simulink model "untitled"  (Simulink 7.3)
settings: Solver=ode45  StartTime=0.0  StopTime=10.0  RelTol=1e-3
values from neighbouring files (symbols this model uses):
  m = 10    [CASEfinder.m]    (also in Example_2ODE_system.m = 9; Example_check_mLyapunov.m; Example_check_mriccati.m)
  R = 100    [Sensitivity_Practice.m]
  w = w_rand_3    [CASEfinder.m]    (also in Example_check_mLyapunov.m; Example_check_mriccati.m; Example_in_Kang_paper.m = 1*rand(length([0:Ts:t_final]),size(Bn,2))'; Road_noise.m = zeros(4,length([0 :Ts: finite_time_of_DOC])))
undefined symbols (not defined in the file or in its folder): DiscIntNeverNeededParam, g, h, Izz, l, lf, lr, ms, mus
settings Model: Creator=SH  LastModifiedBy=SH

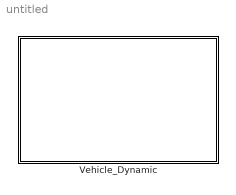
== system untitled ==
  Vehicle_Dynamic : Subsystem
      mask Display: image(imread('V1.jpg'))

== system untitled/Vehicle_Dynamic ==
  Global_position : Subsystem
  Lateral_Dynamic : Subsystem
  Longitudinal_Dynamic : Subsystem
  SlipRatio&SlipAngle : Subsystem
  TireForce : Subsystem
  VerticalForce : Subsystem
  Yaw_Dynamic : Subsystem

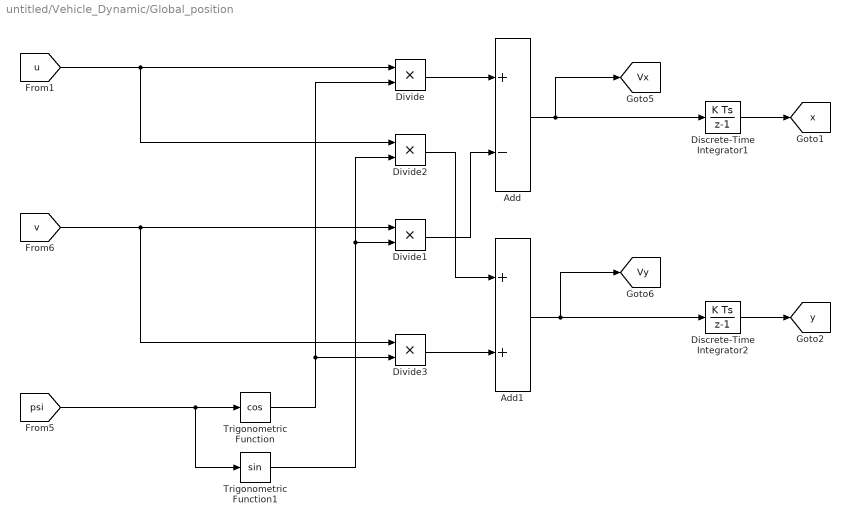
== system untitled/Vehicle_Dynamic/Global_position ==
  Add : Sum  Inputs=+-  OutDataType=fixdt(1, 16)  OutScaling=2^-10
  Add1 : Sum  OutDataType=fixdt(1, 16)  OutScaling=2^-10
  Discrete-Time Integrator1 : DiscreteIntegrator  SampleTime=-1  OutDataType=fixdt(1, 16)  OutScaling=2^0  ICPrevOutput=DiscIntNeverNeededParam  ICPrevScaledInput=DiscIntNeverNeededParam
  Discrete-Time Integrator2 : DiscreteIntegrator  SampleTime=-1  OutDataType=fixdt(1, 16)  OutScaling=2^0  ICPrevOutput=DiscIntNeverNeededParam  ICPrevScaledInput=DiscIntNeverNeededParam
  Divide{,1..3} (4 alike) : Product  Inputs=**  OutDataType=fixdt(1, 16)  OutScaling=2^-10
  Trigonometric Function : Trigonometry  Operator=cos
  Trigonometric Function1 : Trigonometry
  tag scope: Vx=global, Vy=global, x=global, y=global
  wires:
  Add1/1 -> [Vy], Discrete-Time Integrator2/1
  Divide3/1 -> Add1/2
  Divide2/1 -> Add1/1
  Divide1/1 -> Add/2
  Divide/1 -> Add/1
  [v] -> Divide3/1, Divide1/1
  [u] -> Divide2/1, Divide/1
  Discrete-Time Integrator2/1 -> [y]
  Trigonometric Function/1 -> Divide/2, Divide3/2
  Trigonometric Function1/1 -> Divide1/2, Divide2/2
  [psi] -> Trigonometric Function/1, Trigonometric Function1/1
  Discrete-Time Integrator1/1 -> [x]
  Add/1 -> [Vx], Discrete-Time Integrator1/1

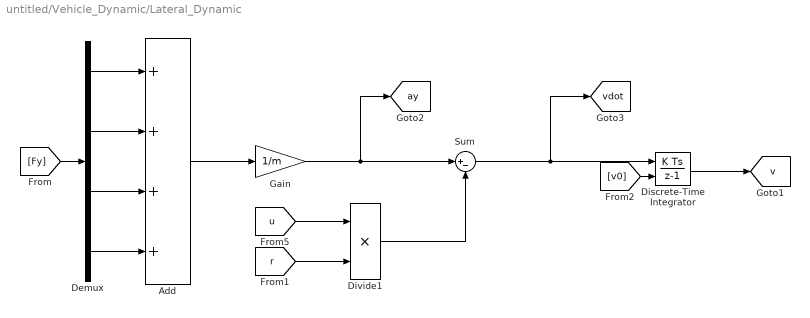
== system untitled/Vehicle_Dynamic/Lateral_Dynamic ==
  Add : Sum  Inputs=++++  OutDataType=fixdt(1, 16)  OutScaling=2^-10
  Demux : Demux
  Discrete-Time Integrator : DiscreteIntegrator  InitialConditionSource=external  SampleTime=-1  OutDataType=fixdt(1, 16)  OutScaling=2^0  ICPrevOutput=DiscIntNeverNeededParam  ICPrevScaledInput=DiscIntNeverNeededParam
  Divide1 : Product  Inputs=**  OutDataType=fixdt(1, 16)  OutScaling=2^-10
  Gain : Gain  Gain=1/m  ParameterDataType=fixdt(1, 16)  ParameterScaling=2^0  OutDataType=fixdt(1, 16)  OutScaling=2^0
  Sum : Sum  Inputs=|+-  OutDataType=fixdt(1, 16)  OutScaling=2^0
  tag scope: ay=global, v=global, vdot=global
  wires:
  Discrete-Time Integrator/1 -> [v]
  [u] -> Divide1/1
  Sum/1 -> Discrete-Time Integrator/1, [vdot]
  Add/1 -> Gain/1
  Gain/1 -> [ay], Sum/1
  [r] -> Divide1/2
  Demux/4 -> Add/4
  Demux/3 -> Add/3
  Demux/2 -> Add/2
  Demux/1 -> Add/1
  [Fy] -> Demux/1
  [v0] -> Discrete-Time Integrator/2
  Divide1/1 -> Sum/2

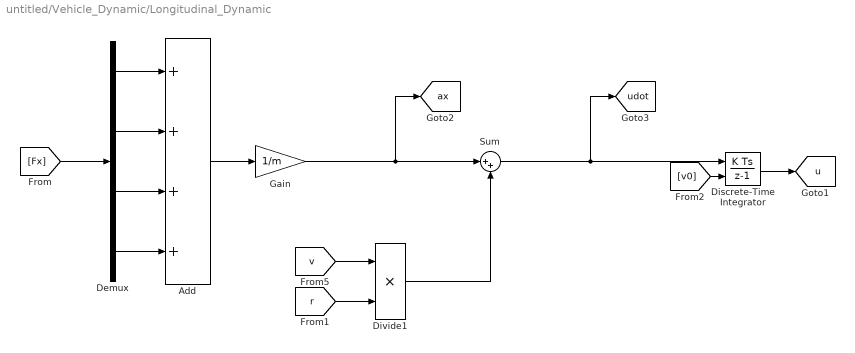
== system untitled/Vehicle_Dynamic/Longitudinal_Dynamic ==
  Add : Sum  Inputs=++++  OutDataType=fixdt(1, 16)  OutScaling=2^-10
  Demux : Demux
  Discrete-Time Integrator : DiscreteIntegrator  InitialConditionSource=external  SampleTime=-1  OutDataType=fixdt(1, 16)  OutScaling=2^0  ICPrevOutput=DiscIntNeverNeededParam  ICPrevScaledInput=DiscIntNeverNeededParam
  Divide1 : Product  Inputs=**  OutDataType=fixdt(1, 16)  OutScaling=2^-10
  Gain : Gain  Gain=1/m  ParameterDataType=fixdt(1, 16)  ParameterScaling=2^0  OutDataType=fixdt(1, 16)  OutScaling=2^0
  Sum : Sum  Inputs=|++  OutDataType=fixdt(1, 16)  OutScaling=2^0
  tag scope: ax=global, u=global, udot=global
  wires:
  Discrete-Time Integrator/1 -> [u]
  Sum/1 -> Discrete-Time Integrator/1, [udot]
  [v] -> Divide1/1
  Add/1 -> Gain/1
  Gain/1 -> [ax], Sum/1
  Demux/4 -> Add/4
  Demux/3 -> Add/3
  Demux/2 -> Add/2
  Demux/1 -> Add/1
  [Fx] -> Demux/1
  [r] -> Divide1/2
  [v0] -> Discrete-Time Integrator/2
  Divide1/1 -> Sum/2

== system untitled/Vehicle_Dynamic/SlipRatio&SlipAngle ==
  Slip_angle : Subsystem
  Slip_ratio : Subsystem
  Tire_Longitudinal_Velocity : Subsystem
  Velocity_at_each_wheel : Subsystem

== system untitled/Vehicle_Dynamic/TireForce ==
  FL : Subsystem
  FR : Subsystem
  RL : Subsystem
  RR : Subsystem

== system untitled/Vehicle_Dynamic/VerticalForce ==
  VerticalForce_FL : Subsystem
  VerticalForce_FR : Subsystem
  VerticalForce_RL : Subsystem
  VerticalForce_RR : Subsystem

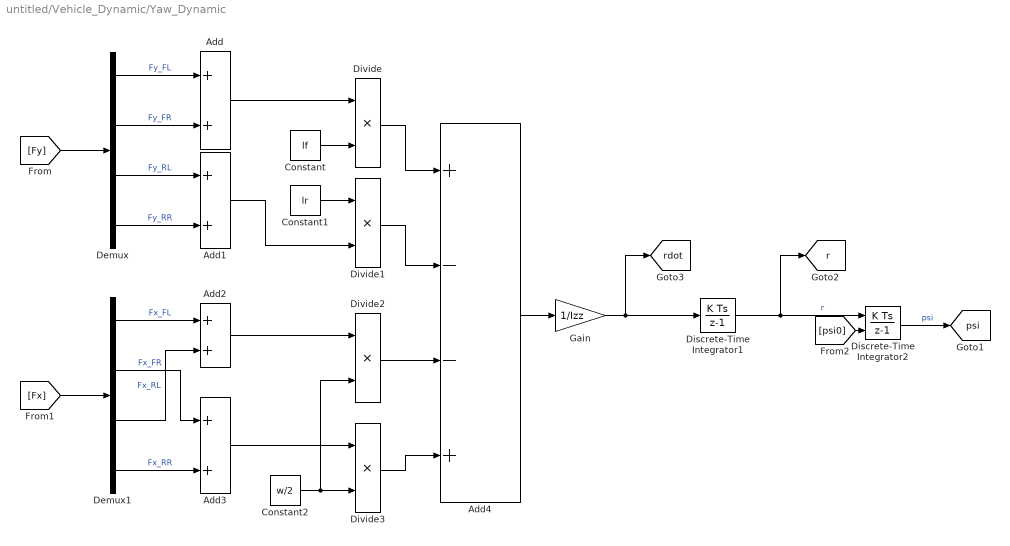
== system untitled/Vehicle_Dynamic/Yaw_Dynamic ==
  Add{,1..3} (4 alike) : Sum  OutDataType=fixdt(1, 16)  OutScaling=2^-10
  Add4 : Sum  Inputs=+--+  OutDataType=fixdt(1, 16)  OutScaling=2^-10
  Constant : Constant  Value=lf  OutDataType=fixdt(1, 16)  OutScaling=2^0
  Constant1 : Constant  Value=lr  OutDataType=fixdt(1, 16)  OutScaling=2^0
  Constant2 : Constant  Value=w/2  OutDataType=fixdt(1, 16)  OutScaling=2^0
  Demux : Demux
  Demux1 : Demux
  Discrete-Time Integrator1 : DiscreteIntegrator  SampleTime=-1  OutDataType=fixdt(1, 16)  OutScaling=2^0  ICPrevOutput=DiscIntNeverNeededParam  ICPrevScaledInput=DiscIntNeverNeededParam
  Discrete-Time Integrator2 : DiscreteIntegrator  InitialConditionSource=external  SampleTime=-1  OutDataType=fixdt(1, 16)  OutScaling=2^0  ICPrevOutput=DiscIntNeverNeededParam  ICPrevScaledInput=DiscIntNeverNeededParam
  Divide{,1..3} (4 alike) : Product  Inputs=**  OutDataType=fixdt(1, 16)  OutScaling=2^-10
  Gain : Gain  Gain=1/Izz  ParameterDataType=fixdt(1, 16)  ParameterScaling=2^0  OutDataType=fixdt(1, 16)  OutScaling=2^0
  tag scope: psi=global, r=global, rdot=global
  wires:
  Add/1 -> Divide/1
  Gain/1 -> Discrete-Time Integrator1/1, [rdot]
  Discrete-Time Integrator1/1 -> Discrete-Time Integrator2/1, [r]  "r"
  Discrete-Time Integrator2/1 -> [psi]  "psi"
  Divide/1 -> Add4/1
  Constant/1 -> Divide/2
  Divide2/1 -> Add4/3
  Divide1/1 -> Add4/2
  Add4/1 -> Gain/1
  Demux/2 -> Add/2  "Fy_FR"
  Demux/1 -> Add/1  "Fy_FL"
  [Fy] -> Demux/1
  [Fx] -> Demux1/1
  [psi0] -> Discrete-Time Integrator2/2
  Demux/3 -> Add1/1  "Fy_RL"
  Demux/4 -> Add1/2  "Fy_RR"
  Constant1/1 -> Divide1/1
  Add1/1 -> Divide1/2
  Divide3/1 -> Add4/4
  Demux1/1 -> Add2/1  "Fx_FL"
  Demux1/4 -> Add3/2  "Fx_RR"
  Add2/1 -> Divide2/1
  Demux1/3 -> Add2/2  "Fx_RL"
  Demux1/2 -> Add3/1  "Fx_FR"
  Add3/1 -> Divide3/1
  Constant2/1 -> Divide3/2, Divide2/2

== system untitled/Vehicle_Dynamic/SlipRatio&SlipAngle/Slip_angle ==
  SlipAngle_FL : Subsystem
  SlipAngle_FR : Subsystem
  SlipAngle_RL : Subsystem
  SlipAngle_RR : Subsystem

== system untitled/Vehicle_Dynamic/SlipRatio&SlipAngle/Slip_ratio ==
  Slipratio_FL : Subsystem
  Slipratio_FR : Subsystem
  Slipratio_RL : Subsystem
  Slipratio_RR : Subsystem

== system untitled/Vehicle_Dynamic/SlipRatio&SlipAngle/Tire_Longitudinal_Velocity ==
  uu_FL : Subsystem
  uu_FR : Subsystem
  uu_RL : Subsystem
  uu_RR : Subsystem

== system untitled/Vehicle_Dynamic/SlipRatio&SlipAngle/Velocity_at_each_wheel ==
  uv_FL : Subsystem
  uv_FR : Subsystem
  uv_RL : Subsystem
  uv_RR : Subsystem

== system untitled/Vehicle_Dynamic/TireForce/FL ==
  SideForce : Subsystem
  TractionForce : Subsystem

== system untitled/Vehicle_Dynamic/TireForce/FR ==
  SideForce : Subsystem
  TractionForce : Subsystem

== system untitled/Vehicle_Dynamic/TireForce/RL ==
  SideForce : Subsystem
  TractionForce : Subsystem

== system untitled/Vehicle_Dynamic/TireForce/RR ==
  SideForce : Subsystem
  TractionForce : Subsystem

== system untitled/Vehicle_Dynamic/VerticalForce/VerticalForce_FL ==
  C.G.Effect : Subsystem
  PitchEffect : Subsystem
  Sum : Sum  Inputs=++-  OutDataType=fixdt(1, 16)  OutScaling=2^0
  TireWeight : Subsystem
  tag scope: Fz_FL=global
  wires:
  Sum/1 -> [Fz_FL]
  TireWeight/1(Out1) -> Sum/1
  C.G.Effect/1(Out1) -> Sum/2
  PitchEffect/1(Out1) -> Sum/3

== system untitled/Vehicle_Dynamic/VerticalForce/VerticalForce_FR ==
  C.G.Effect : Subsystem
  PitchEffect : Subsystem
  Sum : Sum  Inputs=++-  OutDataType=fixdt(1, 16)  OutScaling=2^0
  TireWeight : Subsystem
  tag scope: Fz_FR=global
  wires:
  Sum/1 -> [Fz_FR]
  TireWeight/1(Out1) -> Sum/1
  C.G.Effect/1(Out1) -> Sum/2
  PitchEffect/1(Out1) -> Sum/3

== system untitled/Vehicle_Dynamic/VerticalForce/VerticalForce_RL ==
  C.G.Effect : Subsystem
  PitchEffect : Subsystem
  Sum : Sum  Inputs=+++  OutDataType=fixdt(1, 16)  OutScaling=2^0
  TireWeight : Subsystem
  tag scope: Fz_RL=global
  wires:
  PitchEffect/1(Out1) -> Sum/3
  C.G.Effect/1(Out1) -> Sum/2
  TireWeight/1(Out1) -> Sum/1
  Sum/1 -> [Fz_RL]

== system untitled/Vehicle_Dynamic/VerticalForce/VerticalForce_RR ==
  C.G.Effect : Subsystem
  PitchEffect : Subsystem
  Sum : Sum  Inputs=+++  OutDataType=fixdt(1, 16)  OutScaling=2^0
  TireWeight : Subsystem
  tag scope: Fz_RR=global
  wires:
  PitchEffect/1(Out1) -> Sum/3
  C.G.Effect/1(Out1) -> Sum/2
  TireWeight/1(Out1) -> Sum/1
  Sum/1 -> [Fz_RR]

== system untitled/Vehicle_Dynamic/SlipRatio&SlipAngle/Slip_angle/SlipAngle_FL ==
  Gain : Gain  Gain=pi/180  ParameterDataType=fixdt(1, 16)  ParameterScaling=2^0  OutDataType=fixdt(1, 16)  OutScaling=2^0
  Sum : Sum  Inputs=|+-  OutDataType=fixdt(1, 16)  OutScaling=2^0
  Trigonometric Function : Trigonometry  Operator=atan2
  tag scope: slipA_FL=global
  wires:
  [SA_FL] -> Gain/1
  [u_FL] -> Trigonometric Function/2
  [v_FL] -> Trigonometric Function/1
  Trigonometric Function/1 -> Sum/2
  Gain/1 -> Sum/1
  Sum/1 -> [slipA_FL]

== system untitled/Vehicle_Dynamic/SlipRatio&SlipAngle/Slip_angle/SlipAngle_FR ==
  Gain : Gain  Gain=pi/180  ParameterDataType=fixdt(1, 16)  ParameterScaling=2^0  OutDataType=fixdt(1, 16)  OutScaling=2^0
  Sum : Sum  Inputs=|+-  OutDataType=fixdt(1, 16)  OutScaling=2^0
  Trigonometric Function : Trigonometry  Operator=atan2
  tag scope: slipA_FR=global
  wires:
  Sum/1 -> [slipA_FR]
  Gain/1 -> Sum/1
  Trigonometric Function/1 -> Sum/2
  [v_FR] -> Trigonometric Function/1
  [u_FR] -> Trigonometric Function/2
  [SA_FR] -> Gain/1

== system untitled/Vehicle_Dynamic/SlipRatio&SlipAngle/Slip_angle/SlipAngle_RL ==
  Gain : Gain  Gain=pi/180  ParameterDataType=fixdt(1, 16)  ParameterScaling=2^0  OutDataType=fixdt(1, 16)  OutScaling=2^0
  Sum : Sum  Inputs=|+-  OutDataType=fixdt(1, 16)  OutScaling=2^0
  Trigonometric Function : Trigonometry  Operator=atan2
  tag scope: slipA_RL=global
  wires:
  [SA_RL] -> Gain/1
  [u_RL] -> Trigonometric Function/2
  [v_RL] -> Trigonometric Function/1
  Trigonometric Function/1 -> Sum/2
  Gain/1 -> Sum/1
  Sum/1 -> [slipA_RL]

== system untitled/Vehicle_Dynamic/SlipRatio&SlipAngle/Slip_angle/SlipAngle_RR ==
  Gain : Gain  Gain=pi/180  ParameterDataType=fixdt(1, 16)  ParameterScaling=2^0  OutDataType=fixdt(1, 16)  OutScaling=2^0
  Sum : Sum  Inputs=|+-  OutDataType=fixdt(1, 16)  OutScaling=2^0
  Trigonometric Function : Trigonometry  Operator=atan2
  tag scope: slipA_RR=global
  wires:
  Sum/1 -> [slipA_RR]
  Gain/1 -> Sum/1
  Trigonometric Function/1 -> Sum/2
  [v_RR] -> Trigonometric Function/1
  [u_RR] -> Trigonometric Function/2
  [SA_RR] -> Gain/1

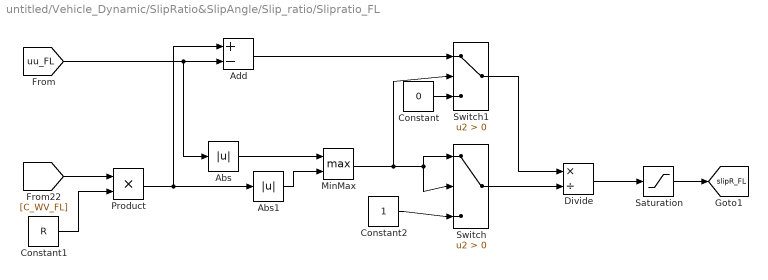
== system untitled/Vehicle_Dynamic/SlipRatio&SlipAngle/Slip_ratio/Slipratio_FL ==
  Abs : Abs  OutDataType=fixdt(1, 16)  OutScaling=2^0
  Abs1 : Abs  OutDataType=fixdt(1, 16)  OutScaling=2^0
  Add : Sum  Inputs=+-  OutDataType=fixdt(1, 16)  OutScaling=2^-10
  Constant : Constant  Value=0  OutDataType=fixdt(1, 16)  OutScaling=2^0
  Constant1 : Constant  Value=R  OutDataType=fixdt(1, 16)  OutScaling=2^0
  Constant2 : Constant  OutDataType=fixdt(1, 16)  OutScaling=2^0
  Divide : Product  Inputs=*/  OutDataType=fixdt(1, 16)  OutScaling=2^-10
  MinMax : MinMax  Function=max  Inputs=2  OutDataType=fixdt(1, 16)  OutScaling=2^0
  Product : Product  OutDataType=fixdt(1, 16)  OutScaling=2^0  RndMeth=Zero
  Saturation : Saturate  UpperLimit=1  LowerLimit=-1  OutDataType=fixdt(1, 16)  OutScaling=2^0
  Switch : Switch  Criteria=u2 > Threshold  OutDataType=fixdt(1, 16)  OutScaling=2^0
  Switch1 : Switch  Criteria=u2 > Threshold  OutDataType=fixdt(1, 16)  OutScaling=2^0
  tag scope: slipR_FL=global
  wires:
  [C_WV_FL] -> Product/1
  Constant1/1 -> Product/2
  Product/1 -> Add/1, Abs1/1
  [uu_FL] -> Add/2, Abs/1
  MinMax/1 -> Switch1/2, Switch/2, Switch/1
  Switch/1 -> Divide/2
  Abs/1 -> MinMax/1
  Abs1/1 -> MinMax/2
  Add/1 -> Switch1/1
  Switch1/1 -> Divide/1
  Constant/1 -> Switch1/3
  Constant2/1 -> Switch/3
  Divide/1 -> Saturation/1
  Saturation/1 -> [slipR_FL]

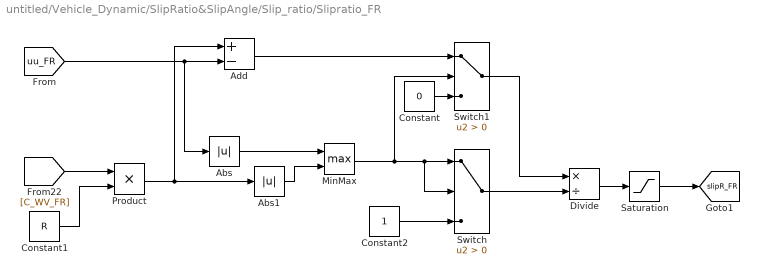
== system untitled/Vehicle_Dynamic/SlipRatio&SlipAngle/Slip_ratio/Slipratio_FR ==
  Abs : Abs  OutDataType=fixdt(1, 16)  OutScaling=2^0
  Abs1 : Abs  OutDataType=fixdt(1, 16)  OutScaling=2^0
  Add : Sum  Inputs=+-  OutDataType=fixdt(1, 16)  OutScaling=2^-10
  Constant : Constant  Value=0  OutDataType=fixdt(1, 16)  OutScaling=2^0
  Constant1 : Constant  Value=R  OutDataType=fixdt(1, 16)  OutScaling=2^0
  Constant2 : Constant  OutDataType=fixdt(1, 16)  OutScaling=2^0
  Divide : Product  Inputs=*/  OutDataType=fixdt(1, 16)  OutScaling=2^-10
  MinMax : MinMax  Function=max  Inputs=2  OutDataType=fixdt(1, 16)  OutScaling=2^0
  Product : Product  OutDataType=fixdt(1, 16)  OutScaling=2^0  RndMeth=Zero
  Saturation : Saturate  UpperLimit=1  LowerLimit=-1  OutDataType=fixdt(1, 16)  OutScaling=2^0
  Switch : Switch  Criteria=u2 > Threshold  OutDataType=fixdt(1, 16)  OutScaling=2^0
  Switch1 : Switch  Criteria=u2 > Threshold  OutDataType=fixdt(1, 16)  OutScaling=2^0
  tag scope: slipR_FR=global
  wires:
  Divide/1 -> Saturation/1
  Constant2/1 -> Switch/3
  Constant/1 -> Switch1/3
  Switch1/1 -> Divide/1
  Add/1 -> Switch1/1
  Abs1/1 -> MinMax/2
  Abs/1 -> MinMax/1
  Switch/1 -> Divide/2
  MinMax/1 -> Switch/1, Switch/2, Switch1/2
  [uu_FR] -> Abs/1, Add/2
  Product/1 -> Abs1/1, Add/1
  Constant1/1 -> Product/2
  [C_WV_FR] -> Product/1
  Saturation/1 -> [slipR_FR]

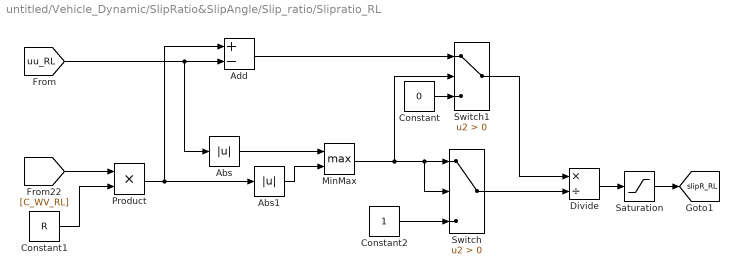
== system untitled/Vehicle_Dynamic/SlipRatio&SlipAngle/Slip_ratio/Slipratio_RL ==
  Abs : Abs  OutDataType=fixdt(1, 16)  OutScaling=2^0
  Abs1 : Abs  OutDataType=fixdt(1, 16)  OutScaling=2^0
  Add : Sum  Inputs=+-  OutDataType=fixdt(1, 16)  OutScaling=2^-10
  Constant : Constant  Value=0  OutDataType=fixdt(1, 16)  OutScaling=2^0
  Constant1 : Constant  Value=R  OutDataType=fixdt(1, 16)  OutScaling=2^0
  Constant2 : Constant  OutDataType=fixdt(1, 16)  OutScaling=2^0
  Divide : Product  Inputs=*/  OutDataType=fixdt(1, 16)  OutScaling=2^-10
  MinMax : MinMax  Function=max  Inputs=2  OutDataType=fixdt(1, 16)  OutScaling=2^0
  Product : Product  OutDataType=fixdt(1, 16)  OutScaling=2^0  RndMeth=Zero
  Saturation : Saturate  UpperLimit=1  LowerLimit=-1  OutDataType=fixdt(1, 16)  OutScaling=2^0
  Switch : Switch  Criteria=u2 > Threshold  OutDataType=fixdt(1, 16)  OutScaling=2^0
  Switch1 : Switch  Criteria=u2 > Threshold  OutDataType=fixdt(1, 16)  OutScaling=2^0
  tag scope: slipR_RL=global
  wires:
  [C_WV_RL] -> Product/1
  Constant1/1 -> Product/2
  [uu_RL] -> Add/2, Abs/1
  MinMax/1 -> Switch1/2, Switch/2, Switch/1
  Switch/1 -> Divide/2
  Abs/1 -> MinMax/1
  Abs1/1 -> MinMax/2
  Add/1 -> Switch1/1
  Switch1/1 -> Divide/1
  Constant/1 -> Switch1/3
  Constant2/1 -> Switch/3
  Divide/1 -> Saturation/1
  Product/1 -> Add/1, Abs1/1
  Saturation/1 -> [slipR_RL]

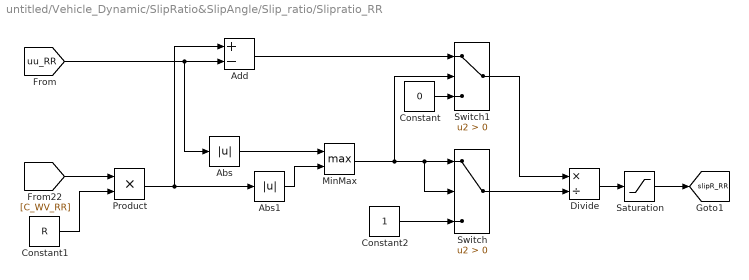
== system untitled/Vehicle_Dynamic/SlipRatio&SlipAngle/Slip_ratio/Slipratio_RR ==
  Abs : Abs  OutDataType=fixdt(1, 16)  OutScaling=2^0
  Abs1 : Abs  OutDataType=fixdt(1, 16)  OutScaling=2^0
  Add : Sum  Inputs=+-  OutDataType=fixdt(1, 16)  OutScaling=2^-10
  Constant : Constant  Value=0  OutDataType=fixdt(1, 16)  OutScaling=2^0
  Constant1 : Constant  Value=R  OutDataType=fixdt(1, 16)  OutScaling=2^0
  Constant2 : Constant  OutDataType=fixdt(1, 16)  OutScaling=2^0
  Divide : Product  Inputs=*/  OutDataType=fixdt(1, 16)  OutScaling=2^-10
  MinMax : MinMax  Function=max  Inputs=2  OutDataType=fixdt(1, 16)  OutScaling=2^0
  Product : Product  OutDataType=fixdt(1, 16)  OutScaling=2^0  RndMeth=Zero
  Saturation : Saturate  UpperLimit=1  LowerLimit=-1  OutDataType=fixdt(1, 16)  OutScaling=2^0
  Switch : Switch  Criteria=u2 > Threshold  OutDataType=fixdt(1, 16)  OutScaling=2^0
  Switch1 : Switch  Criteria=u2 > Threshold  OutDataType=fixdt(1, 16)  OutScaling=2^0
  tag scope: slipR_RR=global
  wires:
  Divide/1 -> Saturation/1
  Constant2/1 -> Switch/3
  Constant/1 -> Switch1/3
  Switch1/1 -> Divide/1
  Add/1 -> Switch1/1
  Abs1/1 -> MinMax/2
  Abs/1 -> MinMax/1
  Switch/1 -> Divide/2
  MinMax/1 -> Switch/1, Switch/2, Switch1/2
  [uu_RR] -> Abs/1, Add/2
  Product/1 -> Abs1/1, Add/1
  Constant1/1 -> Product/2
  [C_WV_RR] -> Product/1
  Saturation/1 -> [slipR_RR]

== system untitled/Vehicle_Dynamic/SlipRatio&SlipAngle/Tire_Longitudinal_Velocity/uu_FL ==
  Gain : Gain  Gain=pi/180  ParameterDataType=fixdt(1, 16)  ParameterScaling=2^0  OutDataType=fixdt(1, 16)  OutScaling=2^0
  Product : Product  OutDataType=fixdt(1, 16)  OutScaling=2^0  RndMeth=Zero
  Product1 : Product  OutDataType=fixdt(1, 16)  OutScaling=2^0  RndMeth=Zero
  Sum : Sum  Inputs=|++  OutDataType=fixdt(1, 16)  OutScaling=2^0
  Trigonometric Function : Trigonometry  Operator=cos
  Trigonometric Function1 : Trigonometry
  tag scope: uu_FL=global
  wires:
  [SA_FL] -> Gain/1
  [u_FL] -> Product/1
  Gain/1 -> Trigonometric Function/1, Trigonometric Function1/1
  Trigonometric Function/1 -> Product/2
  Trigonometric Function1/1 -> Product1/1
  [v_FL] -> Product1/2
  Product/1 -> Sum/1
  Product1/1 -> Sum/2
  Sum/1 -> [uu_FL]

== system untitled/Vehicle_Dynamic/SlipRatio&SlipAngle/Tire_Longitudinal_Velocity/uu_FR ==
  Gain : Gain  Gain=pi/180  ParameterDataType=fixdt(1, 16)  ParameterScaling=2^0  OutDataType=fixdt(1, 16)  OutScaling=2^0
  Product : Product  OutDataType=fixdt(1, 16)  OutScaling=2^0  RndMeth=Zero
  Product1 : Product  OutDataType=fixdt(1, 16)  OutScaling=2^0  RndMeth=Zero
  Sum : Sum  Inputs=|++  OutDataType=fixdt(1, 16)  OutScaling=2^0
  Trigonometric Function : Trigonometry  Operator=cos
  Trigonometric Function1 : Trigonometry
  tag scope: uu_FR=global
  wires:
  [SA_FR] -> Gain/1
  [u_FR] -> Product/1
  Gain/1 -> Trigonometric Function/1, Trigonometric Function1/1
  Trigonometric Function/1 -> Product/2
  Trigonometric Function1/1 -> Product1/1
  [v_FR] -> Product1/2
  Product/1 -> Sum/1
  Product1/1 -> Sum/2
  Sum/1 -> [uu_FR]

== system untitled/Vehicle_Dynamic/SlipRatio&SlipAngle/Tire_Longitudinal_Velocity/uu_RL ==
  Gain : Gain  Gain=pi/180  ParameterDataType=fixdt(1, 16)  ParameterScaling=2^0  OutDataType=fixdt(1, 16)  OutScaling=2^0
  Product : Product  OutDataType=fixdt(1, 16)  OutScaling=2^0  RndMeth=Zero
  Product1 : Product  OutDataType=fixdt(1, 16)  OutScaling=2^0  RndMeth=Zero
  Sum : Sum  Inputs=|++  OutDataType=fixdt(1, 16)  OutScaling=2^0
  Trigonometric Function : Trigonometry  Operator=cos
  Trigonometric Function1 : Trigonometry
  tag scope: uu_RL=global
  wires:
  [SA_RL] -> Gain/1
  [u_RL] -> Product/1
  Gain/1 -> Trigonometric Function/1, Trigonometric Function1/1
  Trigonometric Function/1 -> Product/2
  Trigonometric Function1/1 -> Product1/1
  [v_RL] -> Product1/2
  Product/1 -> Sum/1
  Product1/1 -> Sum/2
  Sum/1 -> [uu_RL]

== system untitled/Vehicle_Dynamic/SlipRatio&SlipAngle/Tire_Longitudinal_Velocity/uu_RR ==
  Gain : Gain  Gain=pi/180  ParameterDataType=fixdt(1, 16)  ParameterScaling=2^0  OutDataType=fixdt(1, 16)  OutScaling=2^0
  Product : Product  OutDataType=fixdt(1, 16)  OutScaling=2^0  RndMeth=Zero
  Product1 : Product  OutDataType=fixdt(1, 16)  OutScaling=2^0  RndMeth=Zero
  Sum : Sum  Inputs=|++  OutDataType=fixdt(1, 16)  OutScaling=2^0
  Trigonometric Function : Trigonometry  Operator=cos
  Trigonometric Function1 : Trigonometry
  tag scope: uu_RR=global
  wires:
  [SA_RR] -> Gain/1
  [u_RR] -> Product/1
  Gain/1 -> Trigonometric Function/1, Trigonometric Function1/1
  Trigonometric Function/1 -> Product/2
  Trigonometric Function1/1 -> Product1/1
  [v_RR] -> Product1/2
  Product/1 -> Sum/1
  Product1/1 -> Sum/2
  Sum/1 -> [uu_RR]

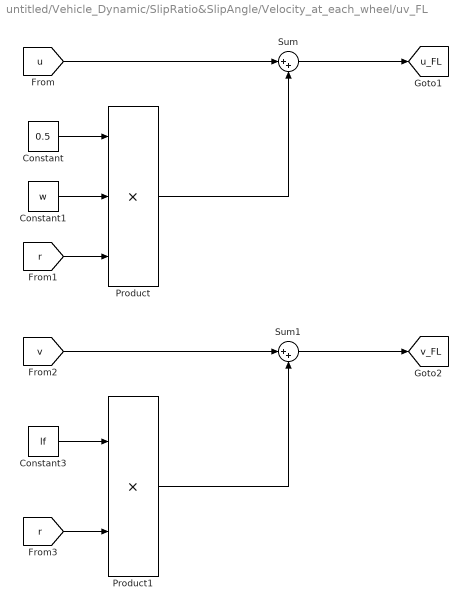
== system untitled/Vehicle_Dynamic/SlipRatio&SlipAngle/Velocity_at_each_wheel/uv_FL ==
  Constant : Constant  Value=0.5  OutDataType=fixdt(1, 16)  OutScaling=2^0
  Constant1 : Constant  Value=w  OutDataType=fixdt(1, 16)  OutScaling=2^0
  Constant3 : Constant  Value=lf  OutDataType=fixdt(1, 16)  OutScaling=2^0
  Product : Product  Inputs=3  OutDataType=fixdt(1, 16)  OutScaling=2^0  RndMeth=Zero
  Product1 : Product  OutDataType=fixdt(1, 16)  OutScaling=2^0  RndMeth=Zero
  Sum : Sum  Inputs=|++  OutDataType=fixdt(1, 16)  OutScaling=2^0
  Sum1 : Sum  Inputs=|++  OutDataType=fixdt(1, 16)  OutScaling=2^0
  tag scope: u_FL=global, v_FL=global
  wires:
  Constant/1 -> Product/1
  Constant1/1 -> Product/2
  [r] -> Product/3
  [u] -> Sum/1
  Product/1 -> Sum/2
  [v] -> Sum1/1
  Product1/1 -> Sum1/2
  Constant3/1 -> Product1/1
  [r] -> Product1/2
  Sum/1 -> [u_FL]
  Sum1/1 -> [v_FL]

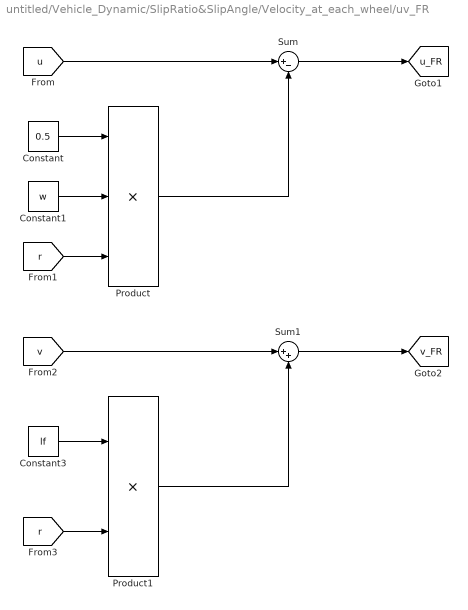
== system untitled/Vehicle_Dynamic/SlipRatio&SlipAngle/Velocity_at_each_wheel/uv_FR ==
  Constant : Constant  Value=0.5  OutDataType=fixdt(1, 16)  OutScaling=2^0
  Constant1 : Constant  Value=w  OutDataType=fixdt(1, 16)  OutScaling=2^0
  Constant3 : Constant  Value=lf  OutDataType=fixdt(1, 16)  OutScaling=2^0
  Product : Product  Inputs=3  OutDataType=fixdt(1, 16)  OutScaling=2^0  RndMeth=Zero
  Product1 : Product  OutDataType=fixdt(1, 16)  OutScaling=2^0  RndMeth=Zero
  Sum : Sum  Inputs=|+-  OutDataType=fixdt(1, 16)  OutScaling=2^0
  Sum1 : Sum  Inputs=|++  OutDataType=fixdt(1, 16)  OutScaling=2^0
  tag scope: u_FR=global, v_FR=global
  wires:
  Sum1/1 -> [v_FR]
  Sum/1 -> [u_FR]
  [r] -> Product1/2
  Constant3/1 -> Product1/1
  Product1/1 -> Sum1/2
  [v] -> Sum1/1
  Product/1 -> Sum/2
  [u] -> Sum/1
  [r] -> Product/3
  Constant1/1 -> Product/2
  Constant/1 -> Product/1

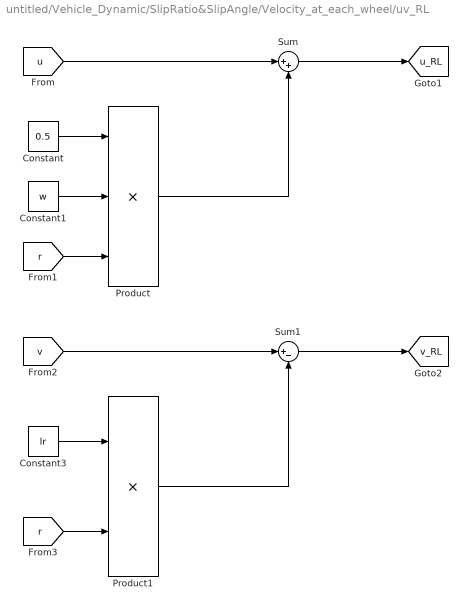
== system untitled/Vehicle_Dynamic/SlipRatio&SlipAngle/Velocity_at_each_wheel/uv_RL ==
  Constant : Constant  Value=0.5  OutDataType=fixdt(1, 16)  OutScaling=2^0
  Constant1 : Constant  Value=w  OutDataType=fixdt(1, 16)  OutScaling=2^0
  Constant3 : Constant  Value=lr  OutDataType=fixdt(1, 16)  OutScaling=2^0
  Product : Product  Inputs=3  OutDataType=fixdt(1, 16)  OutScaling=2^0  RndMeth=Zero
  Product1 : Product  OutDataType=fixdt(1, 16)  OutScaling=2^0  RndMeth=Zero
  Sum : Sum  Inputs=|++  OutDataType=fixdt(1, 16)  OutScaling=2^0
  Sum1 : Sum  Inputs=|+-  OutDataType=fixdt(1, 16)  OutScaling=2^0
  tag scope: u_RL=global, v_RL=global
  wires:
  Constant/1 -> Product/1
  Constant1/1 -> Product/2
  [r] -> Product/3
  [u] -> Sum/1
  Product/1 -> Sum/2
  [v] -> Sum1/1
  Product1/1 -> Sum1/2
  Constant3/1 -> Product1/1
  [r] -> Product1/2
  Sum/1 -> [u_RL]
  Sum1/1 -> [v_RL]

== system untitled/Vehicle_Dynamic/SlipRatio&SlipAngle/Velocity_at_each_wheel/uv_RR ==
  Constant : Constant  Value=0.5  OutDataType=fixdt(1, 16)  OutScaling=2^0
  Constant1 : Constant  Value=w  OutDataType=fixdt(1, 16)  OutScaling=2^0
  Constant3 : Constant  Value=lr  OutDataType=fixdt(1, 16)  OutScaling=2^0
  Product : Product  Inputs=3  OutDataType=fixdt(1, 16)  OutScaling=2^0  RndMeth=Zero
  Product1 : Product  OutDataType=fixdt(1, 16)  OutScaling=2^0  RndMeth=Zero
  Sum : Sum  Inputs=|+-  OutDataType=fixdt(1, 16)  OutScaling=2^0
  Sum1 : Sum  Inputs=|+-  OutDataType=fixdt(1, 16)  OutScaling=2^0
  tag scope: u_RR=global, v_RR=global
  wires:
  Sum1/1 -> [v_RR]
  Sum/1 -> [u_RR]
  [r] -> Product1/2
  Constant3/1 -> Product1/1
  Product1/1 -> Sum1/2
  [v] -> Sum1/1
  Product/1 -> Sum/2
  [u] -> Sum/1
  [r] -> Product/3
  Constant1/1 -> Product/2
  Constant/1 -> Product/1

== system untitled/Vehicle_Dynamic/TireForce/FL/SideForce ==
  Abs : Abs  OutDataType=fixdt(1, 16)  OutScaling=2^0
  Fs (215_55_R17) : Lookup_n-D  BreakpointsForDimension1=[0.5,1,1.5,2,2.5,3,3.5,4,4.5,5,5.5,6,6.5,7,7.5,8,8.5,9,9.5,10,12,14,16,18,20]  BreakpointsForDimension2=[1725,3500,6100,6950,9005]  Table=reshape([444.357,843.546,1162.09,1403.45,1580.72,1707.08,1795.66,1859.6,1893.83,1904.16,1896.19,1875.03,1845.3,1810.95,1775.12,1740.18,1707.8,1678.67,1653.27,1631.62,1574.53,1546.58,1531.91,1523.64,1523.64,894.186,1694.5,2327.41,2800.6,3142.1,3379.93,3542.12,3656.67,3713.24,3724.46,3701.92,3656.45,3597,3531.15,3464.91,3402.12,3345.23,3295.32,3252.61,3216.48,3123.37,3078,3054.18,3040.4,3040.4,1293.54,2452.99,3373.13,4064.18,4565.24,4915.41,5153.78,5319.43,5402.64,5422.23,5395.45,5337.38,5261.2,5177.14,5092.89,5013.56,4942.1,4879.5,4825.96,4780.78,4662.96,4604.6,4573.3,4554.99,4554.99,1601.93,3047.78,4214.48,5111.02,5779.43,6261.69,6599.82,6835.85,6968.31,7019.99,7011.91,6962.7,6887.9,6800.2,6709.15,6621.16,6540.06,6467.91,6405.21,6351.47,6207.67,6133.95,6093.89,6070.17,6070.17,1784.39,3417.9,4780.29,5873.77,6731.16,7385.32,7869.06,8215.23,8439.3,8564.79,8613.61,8605.54,8557.9,8485.17,8398.94,8308.19,8219.02,8135.36,8059.17,7991.56,7798.93,7693.72,7634.76,7599.62,7599.62],25,5)  InputSameDT=on
  Gain : Gain  Gain=180*pi  ParameterDataType=fixdt(1, 16)  ParameterScaling=2^0  OutDataType=fixdt(1, 16)  OutScaling=2^0
  Product : Product  OutDataType=fixdt(1, 16)  OutScaling=2^0  RndMeth=Zero
  Sign : Signum
  tag scope: Fs_FL=global
  wires:
  [slipA_FL] -> Gain/1
  Abs/1 -> Fs (215_55_R17)/1
  [Fz_FL] -> Fs (215_55_R17)/2
  Sign/1 -> Product/1
  Fs (215_55_R17)/1 -> Product/2
  Product/1 -> [Fs_FL]
  Gain/1 -> Abs/1, Sign/1

== system untitled/Vehicle_Dynamic/TireForce/FL/TractionForce ==
  Abs : Abs  OutDataType=fixdt(1, 16)  OutScaling=2^0
  Ft (215_55_R17) : Lookup_n-D  BreakpointsForDimension1=[0.02,0.04,0.06,0.1,0.12,0.14,0.16,0.18,0.2,0.25,0.3,0.4,0.5,0.6,0.7,0.8,0.9,1]  BreakpointsForDimension2=[2105,3995,6120,7900,10100]  Table=reshape([926.741,1701.43,2240.07,2689.78,2729.82,2717.36,2680.7,2634.75,2586.89,2476.95,2388.22,2262.94,2181.64,2125.47,2084.58,2053.55,2029.26,2029.26,1853.48,3402.86,4480.13,5379.54,5459.63,5434.73,5361.4,5269.5,5173.78,4953.9,4776.46,4525.87,4363.28,4250.95,4169.16,4107.12,4058.51,4058.51,2780.22,5104.29,6720.21,8069.32,8189.45,8152.09,8042.1,7904.24,7760.68,7430.85,7164.69,6788.82,6544.93,6376.42,6253.75,6160.67,6087.76,6087.76,3706.97,6805.72,8960.27,10759.1,10919.3,10869.4,10722.8,10539,10347.6,9907.79,9552.92,9051.76,8726.56,8501.91,8338.33,8214.24,8117.01,8117.01,4633.7,8507.15,11200.3,13448.8,13649.1,13586.8,13403.5,13173.7,12934.4,12384.7,11941.1,11314.7,10908.2,10627.4,10422.9,10267.8,10146.3,10146.3],18,5)  InputSameDT=on
  Product : Product  OutDataType=fixdt(1, 16)  OutScaling=2^0  RndMeth=Zero
  Sign : Signum
  tag scope: Ft_FL=global
  wires:
  [slipR_FL] -> Abs/1, Sign/1
  Abs/1 -> Ft (215_55_R17)/1
  [Fz_FL] -> Ft (215_55_R17)/2
  Sign/1 -> Product/1
  Ft (215_55_R17)/1 -> Product/2
  Product/1 -> [Ft_FL]

== system untitled/Vehicle_Dynamic/TireForce/FR/SideForce ==
  Abs : Abs  OutDataType=fixdt(1, 16)  OutScaling=2^0
  Fs (215_55_R17) : Lookup_n-D  BreakpointsForDimension1=[0.5,1,1.5,2,2.5,3,3.5,4,4.5,5,5.5,6,6.5,7,7.5,8,8.5,9,9.5,10,12,14,16,18,20]  BreakpointsForDimension2=[1725,3500,6100,6950,9005]  Table=reshape([444.357,843.546,1162.09,1403.45,1580.72,1707.08,1795.66,1859.6,1893.83,1904.16,1896.19,1875.03,1845.3,1810.95,1775.12,1740.18,1707.8,1678.67,1653.27,1631.62,1574.53,1546.58,1531.91,1523.64,1523.64,894.186,1694.5,2327.41,2800.6,3142.1,3379.93,3542.12,3656.67,3713.24,3724.46,3701.92,3656.45,3597,3531.15,3464.91,3402.12,3345.23,3295.32,3252.61,3216.48,3123.37,3078,3054.18,3040.4,3040.4,1293.54,2452.99,3373.13,4064.18,4565.24,4915.41,5153.78,5319.43,5402.64,5422.23,5395.45,5337.38,5261.2,5177.14,5092.89,5013.56,4942.1,4879.5,4825.96,4780.78,4662.96,4604.6,4573.3,4554.99,4554.99,1601.93,3047.78,4214.48,5111.02,5779.43,6261.69,6599.82,6835.85,6968.31,7019.99,7011.91,6962.7,6887.9,6800.2,6709.15,6621.16,6540.06,6467.91,6405.21,6351.47,6207.67,6133.95,6093.89,6070.17,6070.17,1784.39,3417.9,4780.29,5873.77,6731.16,7385.32,7869.06,8215.23,8439.3,8564.79,8613.61,8605.54,8557.9,8485.17,8398.94,8308.19,8219.02,8135.36,8059.17,7991.56,7798.93,7693.72,7634.76,7599.62,7599.62],25,5)  InputSameDT=on
  Gain : Gain  Gain=180*pi  ParameterDataType=fixdt(1, 16)  ParameterScaling=2^0  OutDataType=fixdt(1, 16)  OutScaling=2^0
  Product : Product  OutDataType=fixdt(1, 16)  OutScaling=2^0  RndMeth=Zero
  Sign : Signum
  tag scope: Fs_FR=global
  wires:
  Gain/1 -> Sign/1, Abs/1
  Product/1 -> [Fs_FR]
  Fs (215_55_R17)/1 -> Product/2
  Sign/1 -> Product/1
  [Fz_FR] -> Fs (215_55_R17)/2
  Abs/1 -> Fs (215_55_R17)/1
  [slipA_FR] -> Gain/1

== system untitled/Vehicle_Dynamic/TireForce/FR/TractionForce ==
  Abs : Abs  OutDataType=fixdt(1, 16)  OutScaling=2^0
  Ft (215_55_R17) : Lookup_n-D  BreakpointsForDimension1=[0.02,0.04,0.06,0.1,0.12,0.14,0.16,0.18,0.2,0.25,0.3,0.4,0.5,0.6,0.7,0.8,0.9,1]  BreakpointsForDimension2=[2105,3995,6120,7900,10100]  Table=reshape([926.741,1701.43,2240.07,2689.78,2729.82,2717.36,2680.7,2634.75,2586.89,2476.95,2388.22,2262.94,2181.64,2125.47,2084.58,2053.55,2029.26,2029.26,1853.48,3402.86,4480.13,5379.54,5459.63,5434.73,5361.4,5269.5,5173.78,4953.9,4776.46,4525.87,4363.28,4250.95,4169.16,4107.12,4058.51,4058.51,2780.22,5104.29,6720.21,8069.32,8189.45,8152.09,8042.1,7904.24,7760.68,7430.85,7164.69,6788.82,6544.93,6376.42,6253.75,6160.67,6087.76,6087.76,3706.97,6805.72,8960.27,10759.1,10919.3,10869.4,10722.8,10539,10347.6,9907.79,9552.92,9051.76,8726.56,8501.91,8338.33,8214.24,8117.01,8117.01,4633.7,8507.15,11200.3,13448.8,13649.1,13586.8,13403.5,13173.7,12934.4,12384.7,11941.1,11314.7,10908.2,10627.4,10422.9,10267.8,10146.3,10146.3],18,5)  InputSameDT=on
  Product : Product  OutDataType=fixdt(1, 16)  OutScaling=2^0  RndMeth=Zero
  Sign : Signum
  tag scope: Ft_FR=global
  wires:
  Product/1 -> [Ft_FR]
  Ft (215_55_R17)/1 -> Product/2
  Sign/1 -> Product/1
  [Fz_FR] -> Ft (215_55_R17)/2
  Abs/1 -> Ft (215_55_R17)/1
  [slipR_FR] -> Sign/1, Abs/1

== system untitled/Vehicle_Dynamic/TireForce/RL/SideForce ==
  Abs : Abs  OutDataType=fixdt(1, 16)  OutScaling=2^0
  Fs (215_55_R17) : Lookup_n-D  BreakpointsForDimension1=[0.5,1,1.5,2,2.5,3,3.5,4,4.5,5,5.5,6,6.5,7,7.5,8,8.5,9,9.5,10,12,14,16,18,20]  BreakpointsForDimension2=[1725,3500,6100,6950,9005]  Table=reshape([444.357,843.546,1162.09,1403.45,1580.72,1707.08,1795.66,1859.6,1893.83,1904.16,1896.19,1875.03,1845.3,1810.95,1775.12,1740.18,1707.8,1678.67,1653.27,1631.62,1574.53,1546.58,1531.91,1523.64,1523.64,894.186,1694.5,2327.41,2800.6,3142.1,3379.93,3542.12,3656.67,3713.24,3724.46,3701.92,3656.45,3597,3531.15,3464.91,3402.12,3345.23,3295.32,3252.61,3216.48,3123.37,3078,3054.18,3040.4,3040.4,1293.54,2452.99,3373.13,4064.18,4565.24,4915.41,5153.78,5319.43,5402.64,5422.23,5395.45,5337.38,5261.2,5177.14,5092.89,5013.56,4942.1,4879.5,4825.96,4780.78,4662.96,4604.6,4573.3,4554.99,4554.99,1601.93,3047.78,4214.48,5111.02,5779.43,6261.69,6599.82,6835.85,6968.31,7019.99,7011.91,6962.7,6887.9,6800.2,6709.15,6621.16,6540.06,6467.91,6405.21,6351.47,6207.67,6133.95,6093.89,6070.17,6070.17,1784.39,3417.9,4780.29,5873.77,6731.16,7385.32,7869.06,8215.23,8439.3,8564.79,8613.61,8605.54,8557.9,8485.17,8398.94,8308.19,8219.02,8135.36,8059.17,7991.56,7798.93,7693.72,7634.76,7599.62,7599.62],25,5)  InputSameDT=on
  Gain : Gain  Gain=180*pi  ParameterDataType=fixdt(1, 16)  ParameterScaling=2^0  OutDataType=fixdt(1, 16)  OutScaling=2^0
  Product : Product  OutDataType=fixdt(1, 16)  OutScaling=2^0  RndMeth=Zero
  Sign : Signum
  tag scope: Fs_RL=global
  wires:
  [slipA_RL] -> Gain/1
  Abs/1 -> Fs (215_55_R17)/1
  [Fz_RL] -> Fs (215_55_R17)/2
  Sign/1 -> Product/1
  Fs (215_55_R17)/1 -> Product/2
  Product/1 -> [Fs_RL]
  Gain/1 -> Abs/1, Sign/1

== system untitled/Vehicle_Dynamic/TireForce/RL/TractionForce ==
  Abs : Abs  OutDataType=fixdt(1, 16)  OutScaling=2^0
  Ft (215_55_R17) : Lookup_n-D  BreakpointsForDimension1=[0.02,0.04,0.06,0.1,0.12,0.14,0.16,0.18,0.2,0.25,0.3,0.4,0.5,0.6,0.7,0.8,0.9,1]  BreakpointsForDimension2=[2105,3995,6120,7900,10100]  Table=reshape([926.741,1701.43,2240.07,2689.78,2729.82,2717.36,2680.7,2634.75,2586.89,2476.95,2388.22,2262.94,2181.64,2125.47,2084.58,2053.55,2029.26,2029.26,1853.48,3402.86,4480.13,5379.54,5459.63,5434.73,5361.4,5269.5,5173.78,4953.9,4776.46,4525.87,4363.28,4250.95,4169.16,4107.12,4058.51,4058.51,2780.22,5104.29,6720.21,8069.32,8189.45,8152.09,8042.1,7904.24,7760.68,7430.85,7164.69,6788.82,6544.93,6376.42,6253.75,6160.67,6087.76,6087.76,3706.97,6805.72,8960.27,10759.1,10919.3,10869.4,10722.8,10539,10347.6,9907.79,9552.92,9051.76,8726.56,8501.91,8338.33,8214.24,8117.01,8117.01,4633.7,8507.15,11200.3,13448.8,13649.1,13586.8,13403.5,13173.7,12934.4,12384.7,11941.1,11314.7,10908.2,10627.4,10422.9,10267.8,10146.3,10146.3],18,5)  InputSameDT=on
  Product : Product  OutDataType=fixdt(1, 16)  OutScaling=2^0  RndMeth=Zero
  Sign : Signum
  tag scope: Ft_RL=global
  wires:
  [slipR_RL] -> Abs/1, Sign/1
  Abs/1 -> Ft (215_55_R17)/1
  [Fz_RL] -> Ft (215_55_R17)/2
  Sign/1 -> Product/1
  Ft (215_55_R17)/1 -> Product/2
  Product/1 -> [Ft_RL]

== system untitled/Vehicle_Dynamic/TireForce/RR/SideForce ==
  Abs : Abs  OutDataType=fixdt(1, 16)  OutScaling=2^0
  Fs (215_55_R17) : Lookup_n-D  BreakpointsForDimension1=[0.5,1,1.5,2,2.5,3,3.5,4,4.5,5,5.5,6,6.5,7,7.5,8,8.5,9,9.5,10,12,14,16,18,20]  BreakpointsForDimension2=[1725,3500,6100,6950,9005]  Table=reshape([444.357,843.546,1162.09,1403.45,1580.72,1707.08,1795.66,1859.6,1893.83,1904.16,1896.19,1875.03,1845.3,1810.95,1775.12,1740.18,1707.8,1678.67,1653.27,1631.62,1574.53,1546.58,1531.91,1523.64,1523.64,894.186,1694.5,2327.41,2800.6,3142.1,3379.93,3542.12,3656.67,3713.24,3724.46,3701.92,3656.45,3597,3531.15,3464.91,3402.12,3345.23,3295.32,3252.61,3216.48,3123.37,3078,3054.18,3040.4,3040.4,1293.54,2452.99,3373.13,4064.18,4565.24,4915.41,5153.78,5319.43,5402.64,5422.23,5395.45,5337.38,5261.2,5177.14,5092.89,5013.56,4942.1,4879.5,4825.96,4780.78,4662.96,4604.6,4573.3,4554.99,4554.99,1601.93,3047.78,4214.48,5111.02,5779.43,6261.69,6599.82,6835.85,6968.31,7019.99,7011.91,6962.7,6887.9,6800.2,6709.15,6621.16,6540.06,6467.91,6405.21,6351.47,6207.67,6133.95,6093.89,6070.17,6070.17,1784.39,3417.9,4780.29,5873.77,6731.16,7385.32,7869.06,8215.23,8439.3,8564.79,8613.61,8605.54,8557.9,8485.17,8398.94,8308.19,8219.02,8135.36,8059.17,7991.56,7798.93,7693.72,7634.76,7599.62,7599.62],25,5)  InputSameDT=on
  Gain : Gain  Gain=180*pi  ParameterDataType=fixdt(1, 16)  ParameterScaling=2^0  OutDataType=fixdt(1, 16)  OutScaling=2^0
  Product : Product  OutDataType=fixdt(1, 16)  OutScaling=2^0  RndMeth=Zero
  Sign : Signum
  tag scope: Fs_RR=global
  wires:
  Gain/1 -> Sign/1, Abs/1
  Product/1 -> [Fs_RR]
  Fs (215_55_R17)/1 -> Product/2
  Sign/1 -> Product/1
  [Fz_RR] -> Fs (215_55_R17)/2
  Abs/1 -> Fs (215_55_R17)/1
  [slipA_RR] -> Gain/1

== system untitled/Vehicle_Dynamic/TireForce/RR/TractionForce ==
  Abs : Abs  OutDataType=fixdt(1, 16)  OutScaling=2^0
  Ft (215_55_R17) : Lookup_n-D  BreakpointsForDimension1=[0.02,0.04,0.06,0.1,0.12,0.14,0.16,0.18,0.2,0.25,0.3,0.4,0.5,0.6,0.7,0.8,0.9,1]  BreakpointsForDimension2=[2105,3995,6120,7900,10100]  Table=reshape([926.741,1701.43,2240.07,2689.78,2729.82,2717.36,2680.7,2634.75,2586.89,2476.95,2388.22,2262.94,2181.64,2125.47,2084.58,2053.55,2029.26,2029.26,1853.48,3402.86,4480.13,5379.54,5459.63,5434.73,5361.4,5269.5,5173.78,4953.9,4776.46,4525.87,4363.28,4250.95,4169.16,4107.12,4058.51,4058.51,2780.22,5104.29,6720.21,8069.32,8189.45,8152.09,8042.1,7904.24,7760.68,7430.85,7164.69,6788.82,6544.93,6376.42,6253.75,6160.67,6087.76,6087.76,3706.97,6805.72,8960.27,10759.1,10919.3,10869.4,10722.8,10539,10347.6,9907.79,9552.92,9051.76,8726.56,8501.91,8338.33,8214.24,8117.01,8117.01,4633.7,8507.15,11200.3,13448.8,13649.1,13586.8,13403.5,13173.7,12934.4,12384.7,11941.1,11314.7,10908.2,10627.4,10422.9,10267.8,10146.3,10146.3],18,5)  InputSameDT=on
  Product : Product  OutDataType=fixdt(1, 16)  OutScaling=2^0  RndMeth=Zero
  Sign : Signum
  tag scope: Ft_RR=global
  wires:
  Product/1 -> [Ft_RR]
  Ft (215_55_R17)/1 -> Product/2
  Sign/1 -> Product/1
  [Fz_RR] -> Ft (215_55_R17)/2
  Abs/1 -> Ft (215_55_R17)/1
  [slipR_RR] -> Sign/1, Abs/1

== system untitled/Vehicle_Dynamic/VerticalForce/VerticalForce_FL/C.G.Effect ==
  Constant3 : Constant  Value=0.5  OutDataType=fixdt(1, 16)  OutScaling=2^0
  Constant4 : Constant  Value=ms  OutDataType=fixdt(1, 16)  OutScaling=2^0
  Constant5 : Constant  Value=g  OutDataType=fixdt(1, 16)  OutScaling=2^0
  Constant6 : Constant  Value=lr  OutDataType=fixdt(1, 16)  OutScaling=2^0
  Constant7 : Constant  Value=l  OutDataType=fixdt(1, 16)  OutScaling=2^0
  Divide : Product  Inputs=****/  OutDataType=fixdt(1, 16)  OutScaling=2^-10
  Out1 : Outport  OutDataType=fixdt(1, 16)  OutScaling=2^0
  wires:
  Constant3/1 -> Divide/1
  Constant4/1 -> Divide/2
  Constant5/1 -> Divide/3
  Constant6/1 -> Divide/4
  Constant7/1 -> Divide/5
  Divide/1 -> Out1/1

== system untitled/Vehicle_Dynamic/VerticalForce/VerticalForce_FL/PitchEffect ==
  Constant11 : Constant  Value=h  OutDataType=fixdt(1, 16)  OutScaling=2^0
  Constant12 : Constant  Value=l  OutDataType=fixdt(1, 16)  OutScaling=2^0
  Constant8 : Constant  Value=0.5  OutDataType=fixdt(1, 16)  OutScaling=2^0
  Constant9 : Constant  Value=m  OutDataType=fixdt(1, 16)  OutScaling=2^0
  Divide1 : Product  Inputs=****/  OutDataType=fixdt(1, 16)  OutScaling=2^-10
  Out1 : Outport  OutDataType=fixdt(1, 16)  OutScaling=2^0
  wires:
  Constant8/1 -> Divide1/1
  Constant9/1 -> Divide1/2
  [ax] -> Divide1/3
  Constant11/1 -> Divide1/4
  Constant12/1 -> Divide1/5
  Divide1/1 -> Out1/1

== system untitled/Vehicle_Dynamic/VerticalForce/VerticalForce_FL/TireWeight ==
  Constant : Constant  Value=0.25  OutDataType=fixdt(1, 16)  OutScaling=2^0
  Constant1 : Constant  Value=mus  OutDataType=fixdt(1, 16)  OutScaling=2^0
  Constant2 : Constant  Value=g  OutDataType=fixdt(1, 16)  OutScaling=2^0
  Product : Product  Inputs=3  OutDataType=fixdt(1, 16)  OutScaling=2^0  RndMeth=Zero
  Out1 : Outport  OutDataType=fixdt(1, 16)  OutScaling=2^0
  wires:
  Constant/1 -> Product/1
  Constant1/1 -> Product/2
  Constant2/1 -> Product/3
  Product/1 -> Out1/1

== system untitled/Vehicle_Dynamic/VerticalForce/VerticalForce_FR/C.G.Effect ==
  Constant3 : Constant  Value=0.5  OutDataType=fixdt(1, 16)  OutScaling=2^0
  Constant4 : Constant  Value=ms  OutDataType=fixdt(1, 16)  OutScaling=2^0
  Constant5 : Constant  Value=g  OutDataType=fixdt(1, 16)  OutScaling=2^0
  Constant6 : Constant  Value=lr  OutDataType=fixdt(1, 16)  OutScaling=2^0
  Constant7 : Constant  Value=l  OutDataType=fixdt(1, 16)  OutScaling=2^0
  Divide : Product  Inputs=****/  OutDataType=fixdt(1, 16)  OutScaling=2^-10
  Out1 : Outport  OutDataType=fixdt(1, 16)  OutScaling=2^0
  wires:
  Constant3/1 -> Divide/1
  Constant4/1 -> Divide/2
  Constant5/1 -> Divide/3
  Constant6/1 -> Divide/4
  Constant7/1 -> Divide/5
  Divide/1 -> Out1/1

== system untitled/Vehicle_Dynamic/VerticalForce/VerticalForce_FR/PitchEffect ==
  Constant11 : Constant  Value=h  OutDataType=fixdt(1, 16)  OutScaling=2^0
  Constant12 : Constant  Value=l  OutDataType=fixdt(1, 16)  OutScaling=2^0
  Constant8 : Constant  Value=0.5  OutDataType=fixdt(1, 16)  OutScaling=2^0
  Constant9 : Constant  Value=m  OutDataType=fixdt(1, 16)  OutScaling=2^0
  Divide1 : Product  Inputs=****/  OutDataType=fixdt(1, 16)  OutScaling=2^-10
  Out1 : Outport  OutDataType=fixdt(1, 16)  OutScaling=2^0
  wires:
  Constant8/1 -> Divide1/1
  Constant9/1 -> Divide1/2
  [ax] -> Divide1/3
  Constant11/1 -> Divide1/4
  Constant12/1 -> Divide1/5
  Divide1/1 -> Out1/1

== system untitled/Vehicle_Dynamic/VerticalForce/VerticalForce_FR/TireWeight ==
  Constant : Constant  Value=0.25  OutDataType=fixdt(1, 16)  OutScaling=2^0
  Constant1 : Constant  Value=mus  OutDataType=fixdt(1, 16)  OutScaling=2^0
  Constant2 : Constant  Value=g  OutDataType=fixdt(1, 16)  OutScaling=2^0
  Product : Product  Inputs=3  OutDataType=fixdt(1, 16)  OutScaling=2^0  RndMeth=Zero
  Out1 : Outport  OutDataType=fixdt(1, 16)  OutScaling=2^0
  wires:
  Constant/1 -> Product/1
  Constant1/1 -> Product/2
  Constant2/1 -> Product/3
  Product/1 -> Out1/1

== system untitled/Vehicle_Dynamic/VerticalForce/VerticalForce_RL/C.G.Effect ==
  Constant3 : Constant  Value=0.5  OutDataType=fixdt(1, 16)  OutScaling=2^0
  Constant4 : Constant  Value=ms  OutDataType=fixdt(1, 16)  OutScaling=2^0
  Constant5 : Constant  Value=g  OutDataType=fixdt(1, 16)  OutScaling=2^0
  Constant6 : Constant  Value=lf  OutDataType=fixdt(1, 16)  OutScaling=2^0
  Constant7 : Constant  Value=l  OutDataType=fixdt(1, 16)  OutScaling=2^0
  Divide : Product  Inputs=****/  OutDataType=fixdt(1, 16)  OutScaling=2^-10
  Out1 : Outport  OutDataType=fixdt(1, 16)  OutScaling=2^0
  wires:
  Divide/1 -> Out1/1
  Constant7/1 -> Divide/5
  Constant6/1 -> Divide/4
  Constant5/1 -> Divide/3
  Constant4/1 -> Divide/2
  Constant3/1 -> Divide/1

== system untitled/Vehicle_Dynamic/VerticalForce/VerticalForce_RL/PitchEffect ==
  Constant11 : Constant  Value=h  OutDataType=fixdt(1, 16)  OutScaling=2^0
  Constant12 : Constant  Value=l  OutDataType=fixdt(1, 16)  OutScaling=2^0
  Constant8 : Constant  Value=0.5  OutDataType=fixdt(1, 16)  OutScaling=2^0
  Constant9 : Constant  Value=m  OutDataType=fixdt(1, 16)  OutScaling=2^0
  Divide1 : Product  Inputs=****/  OutDataType=fixdt(1, 16)  OutScaling=2^-10
  Out1 : Outport  OutDataType=fixdt(1, 16)  OutScaling=2^0
  wires:
  Divide1/1 -> Out1/1
  Constant12/1 -> Divide1/5
  Constant11/1 -> Divide1/4
  [ax] -> Divide1/3
  Constant9/1 -> Divide1/2
  Constant8/1 -> Divide1/1

== system untitled/Vehicle_Dynamic/VerticalForce/VerticalForce_RL/TireWeight ==
  Constant : Constant  Value=0.25  OutDataType=fixdt(1, 16)  OutScaling=2^0
  Constant1 : Constant  Value=mus  OutDataType=fixdt(1, 16)  OutScaling=2^0
  Constant2 : Constant  Value=g  OutDataType=fixdt(1, 16)  OutScaling=2^0
  Product : Product  Inputs=3  OutDataType=fixdt(1, 16)  OutScaling=2^0  RndMeth=Zero
  Out1 : Outport  OutDataType=fixdt(1, 16)  OutScaling=2^0
  wires:
  Product/1 -> Out1/1
  Constant2/1 -> Product/3
  Constant1/1 -> Product/2
  Constant/1 -> Product/1

== system untitled/Vehicle_Dynamic/VerticalForce/VerticalForce_RR/C.G.Effect ==
  Constant3 : Constant  Value=0.5  OutDataType=fixdt(1, 16)  OutScaling=2^0
  Constant4 : Constant  Value=ms  OutDataType=fixdt(1, 16)  OutScaling=2^0
  Constant5 : Constant  Value=g  OutDataType=fixdt(1, 16)  OutScaling=2^0
  Constant6 : Constant  Value=lf  OutDataType=fixdt(1, 16)  OutScaling=2^0
  Constant7 : Constant  Value=l  OutDataType=fixdt(1, 16)  OutScaling=2^0
  Divide : Product  Inputs=****/  OutDataType=fixdt(1, 16)  OutScaling=2^-10
  Out1 : Outport  OutDataType=fixdt(1, 16)  OutScaling=2^0
  wires:
  Divide/1 -> Out1/1
  Constant7/1 -> Divide/5
  Constant6/1 -> Divide/4
  Constant5/1 -> Divide/3
  Constant4/1 -> Divide/2
  Constant3/1 -> Divide/1

== system untitled/Vehicle_Dynamic/VerticalForce/VerticalForce_RR/PitchEffect ==
  Constant11 : Constant  Value=h  OutDataType=fixdt(1, 16)  OutScaling=2^0
  Constant12 : Constant  Value=l  OutDataType=fixdt(1, 16)  OutScaling=2^0
  Constant8 : Constant  Value=0.5  OutDataType=fixdt(1, 16)  OutScaling=2^0
  Constant9 : Constant  Value=m  OutDataType=fixdt(1, 16)  OutScaling=2^0
  Divide1 : Product  Inputs=****/  OutDataType=fixdt(1, 16)  OutScaling=2^-10
  Out1 : Outport  OutDataType=fixdt(1, 16)  OutScaling=2^0
  wires:
  Divide1/1 -> Out1/1
  Constant12/1 -> Divide1/5
  Constant11/1 -> Divide1/4
  [ax] -> Divide1/3
  Constant9/1 -> Divide1/2
  Constant8/1 -> Divide1/1

== system untitled/Vehicle_Dynamic/VerticalForce/VerticalForce_RR/TireWeight ==
  Constant : Constant  Value=0.25  OutDataType=fixdt(1, 16)  OutScaling=2^0
  Constant1 : Constant  Value=mus  OutDataType=fixdt(1, 16)  OutScaling=2^0
  Constant2 : Constant  Value=g  OutDataType=fixdt(1, 16)  OutScaling=2^0
  Product : Product  Inputs=3  OutDataType=fixdt(1, 16)  OutScaling=2^0  RndMeth=Zero
  Out1 : Outport  OutDataType=fixdt(1, 16)  OutScaling=2^0
  wires:
  Product/1 -> Out1/1
  Constant2/1 -> Product/3
  Constant1/1 -> Product/2
  Constant/1 -> Product/1
